simulink library "IP_MASTER_backup20190216"  (Simulink 8.6)
settings: Solver=ode45  StartTime=0.0  StopTime=10.0  RelTol=1e-3
libraries: cdsFilt x19, cdsEpicsOut x14, cdsFiltCtrl x12, cdsTP x6, cdsMuxMatrix x3, cdsEpicsIn x3, cdsFunctionCall x1, SIXOSEM_F_WD_AC_MASTER x1, SIXOSEM_F_STAGE_MASTER x1
(part 1 of 4)
settings Model: Creator=controls  LastModifiedBy=controls

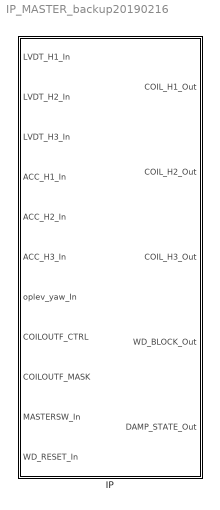
== system IP_MASTER_backup20190216 ==
  IP : Subsystem

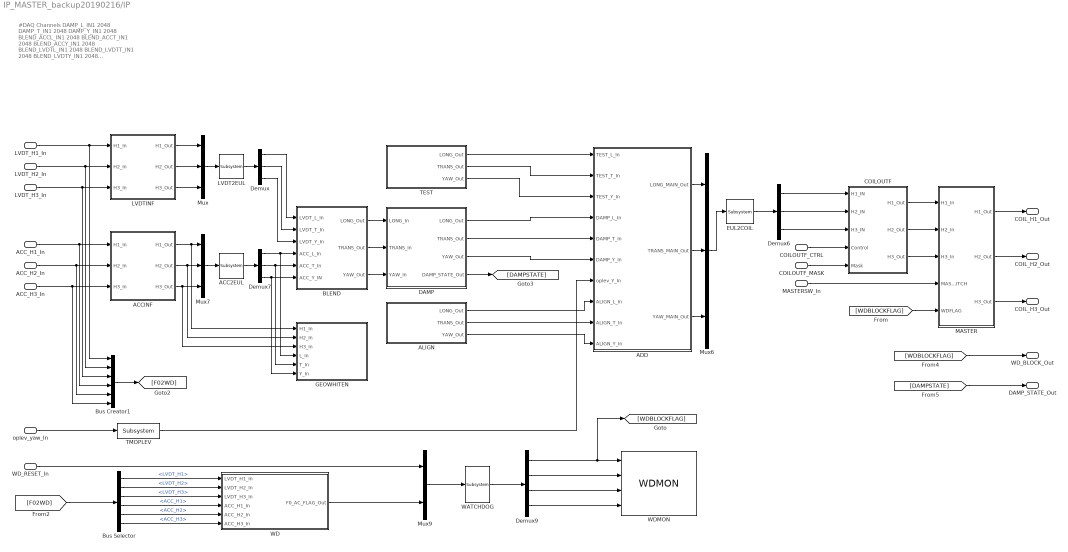
== system IP_MASTER_backup20190216/IP ==
  note: #DAQ Channels
      | DAMP_L_IN1 2048
      | DAMP_T_IN1 2048
      | DAMP_Y_IN1 2048
      | BLEND_ACCL_IN1 2048
      | BLEND_ACCT_IN1 2048
      | BLEND_ACCY_IN1 2048
      | BLEND_LVDTL_IN1 2048
      | BLEND_LVDTT_IN1 2048
      | BLEND_LVDTY_IN1 2048
      | GEOWHITEN_L_OUT 2048
      | GEOWHITEN_T_OUT 2048
      | GEOWHITEN_Y_OUT 2048
  LVDT_H1_In : Inport
  LVDT_H2_In : Inport  Port=2
  LVDT_H3_In : Inport  Port=3
  ACC_H1_In : Inport  Port=4
  ACC_H2_In : Inport  Port=5
  ACC_H3_In : Inport  Port=6
  oplev_yaw_In : Inport  Port=7
  COILOUTF_CTRL : Inport  Port=8
  COILOUTF_MASK : Inport  Port=9
  MASTERSW_In : Inport  Port=10
  WD_RESET_In : Inport  Port=11
  ACC2EUL : cdsMuxMatrix/Subsystem  Tag=cdsMuxMatrix  Description=|
      | ADL=SUS_INMATRIX.adl
      | SCRIPT=generate_KisselButton.py 4 5 #CHANNEL# > #TARGET_DIR#/#FULL_PART_NAME#_KB.adl
      settings: AttributesFormatString=%<Tag>
  ACCINF : Subsystem
  ADD : Subsystem
  ALIGN : Subsystem
  BLEND : Subsystem
  Bus Creator1 : BusCreator  Inputs='LVDT_H1','LVDT_H2','LVDT_H3','ACC_H1','ACC_H2','ACC_H3'
  Bus Selector : BusSelector  OutputSignals=LVDT_H1,LVDT_H2,LVDT_H3,ACC_H1,ACC_H2,ACC_H3
  COILOUTF : Subsystem
  DAMP : Subsystem
  Demux : Demux  Outputs=3
  Demux6 : Demux  Outputs=3
  Demux7 : Demux  Outputs=3
  Demux9 : Demux
  EUL2COIL : cdsMuxMatrix/Subsystem  Tag=cdsMuxMatrix  Description=|
      | ADL=SUS_INMATRIX.adl
      | SCRIPT=generate_KisselButton.py 4 5 #CHANNEL# > #TARGET_DIR#/#FULL_PART_NAME#_KB.adl
      settings: AttributesFormatString=%<Tag>
  GEOWHITEN : Subsystem
  LVDT2EUL : cdsMuxMatrix/Subsystem  Tag=cdsMuxMatrix  Description=|
      | ADL=SUS_INMATRIX.adl
      | SCRIPT=generate_KisselButton.py 4 5 #CHANNEL# > #TARGET_DIR#/#FULL_PART_NAME#_KB.adl
      settings: AttributesFormatString=%<Tag>
  LVDTINF : Subsystem
  MASTER : Subsystem
  Mux : Mux  Inputs=3
  Mux6 : Mux  Inputs=3
  Mux7 : Mux  Inputs=3
  Mux9 : Mux  Inputs=2
  TEST : Subsystem
  TMOPLEV : cdsFilt/Subsystem  Tag=cdsFilt  Description=|
      | Purpose:                                                                                                                                                                                                                                  
      | Standard CDS IIR filter module.                                                                                                                                                                                                           
      |                                                                                                                                                                                                                                           
      | Operation:                                                                                                                                                                                                                                
      | Consists of 10 second order section IIR filters, plus a ramped gain stage. In FE code, also provides pre-defined test points and excitation channel inputs. The filter coefficients are defined in the LIGO system using the 'foton' tool.
      |                                                                                                                                                                                                                                           
      | Usage:                                                                                                                                                                                                                                    
      | Name the part with the desired filter module name.
      settings: AttributesFormatString=%<Tag>
  WATCHDOG : cdsFunctionCall/Subsystem  Tag=cdsFunctionCall  Description=inline OSEMWATCHDOG /opt/rtcds/userapps/release/vis/common/src/WATCHDOG.c
      settings: AttributesFormatString=%<Tag>\n%<Description>
  WD : Subsystem
  WDMON : SIXOSEM_F_STAGE_MASTER/SIXOSEM_F_STAGE_MASTER/WDMON
  COIL_H1_Out : Outport
  COIL_H2_Out : Outport  Port=2
  COIL_H3_Out : Outport  Port=3
  WD_BLOCK_Out : Outport  Port=4
  DAMP_STATE_Out : Outport  Port=5
  wires:
  LVDTINF/1(H1_Out) -> Mux/1
  LVDTINF/2(H2_Out) -> Mux/2
  LVDTINF/3(H3_Out) -> Mux/3
  Mux/1 -> LVDT2EUL/1
  LVDT2EUL/1 -> Demux/1
  Mux7/1 -> ACC2EUL/1
  ACCINF/1(H1_Out) -> GEOWHITEN/1(H1_In), Mux7/1
  ACCINF/3(H3_Out) -> GEOWHITEN/3(H3_In), Mux7/3
  ACCINF/2(H2_Out) -> GEOWHITEN/2(H2_In), Mux7/2
  ACC2EUL/1 -> Demux7/1
  Demux/1 -> BLEND/1(LVDT_L_In)
  Demux/2 -> BLEND/2(LVDT_T_In)
  Demux/3 -> BLEND/3(LVDT_Y_In)
  Demux7/1 -> GEOWHITEN/4(L_In), BLEND/4(ACC_L_In)
  Demux7/2 -> GEOWHITEN/5(T_In), BLEND/5(ACC_T_In)
  Demux7/3 -> GEOWHITEN/6(Y_In), BLEND/6(ACC_Y_IN)
  ADD/1(LONG_MAIN_Out) -> Mux6/1
  ADD/2(TRANS_MAIN_Out) -> Mux6/2
  ADD/3(YAW_MAIN_Out) -> Mux6/3
  Mux6/1 -> EUL2COIL/1
  EUL2COIL/1 -> Demux6/1
  Demux6/1 -> COILOUTF/1(H1_IN)
  Demux6/2 -> COILOUTF/2(H2_IN)
  Demux6/3 -> COILOUTF/3(H3_IN)
  MASTER/1(H1_Out) -> COIL_H1_Out/1
  MASTER/2(H2_Out) -> COIL_H2_Out/1
  MASTER/3(H3_Out) -> COIL_H3_Out/1
  COILOUTF/1(H1_Out) -> MASTER/1(H1_In)
  COILOUTF/2(H2_Out) -> MASTER/2(H2_In)
  COILOUTF/3(H3_Out) -> MASTER/3(H3_In)
  MASTERSW_In/1 -> MASTER/4(MASTERSWITCH)
  WD_RESET_In/1 -> Mux9/1
  WD/1(F0_AC_FLAG_Out) -> Mux9/2
  [F02WD] -> Bus Selector/1
  Bus Selector/1 -> WD/1(LVDT_H1_In)  "<LVDT_H1>"
  Bus Selector/2 -> WD/2(LVDT_H2_In)  "<LVDT_H2>"
  Bus Selector/3 -> WD/3(LVDT_H3_In)  "<LVDT_H3>"
  Bus Selector/4 -> WD/4(ACC_H1_In)  "<ACC_H1>"
  Bus Selector/6 -> WD/6(ACC_H3_In)  "<ACC_H3>"
  Bus Selector/5 -> WD/5(ACC_H2_In)  "<ACC_H2>"
  Demux9/1 -> [WDBLOCKFLAG], WDMON/1
  Demux9/2 -> WDMON/2
  Demux9/3 -> WDMON/3
  Demux9/4 -> WDMON/4
  Mux9/1 -> WATCHDOG/1
  WATCHDOG/1 -> Demux9/1
  LVDT_H1_In/1 -> Bus Creator1/1, LVDTINF/1(H1_In)
  LVDT_H2_In/1 -> Bus Creator1/2, LVDTINF/2(H2_In)
  LVDT_H3_In/1 -> Bus Creator1/3, LVDTINF/3(H3_In)
  ACC_H1_In/1 -> Bus Creator1/4, ACCINF/1(H1_In)
  ACC_H2_In/1 -> Bus Creator1/5, ACCINF/2(H2_In)
  ACC_H3_In/1 -> Bus Creator1/6, ACCINF/3(H3_In)
  Bus Creator1/1 -> [F02WD]
  [WDBLOCKFLAG] -> MASTER/5(WDFLAG)
  BLEND/1(LONG_Out) -> DAMP/1(LONG_In)
  BLEND/2(TRANS_Out) -> DAMP/2(TRANS_In)
  BLEND/3(YAW_Out) -> DAMP/3(YAW_In)
  DAMP/4(DAMP_STATE_Out) -> [DAMPSTATE]
  TEST/1(LONG_Out) -> ADD/1(TEST_L_In)
  TEST/2(TRANS_Out) -> ADD/2(TEST_T_In)
  TEST/3(YAW_Out) -> ADD/3(TEST_Y_In)
  DAMP/1(LONG_Out) -> ADD/4(DAMP_L_In)
  DAMP/2(TRANS_Out) -> ADD/5(DAMP_T_In)
  DAMP/3(YAW_Out) -> ADD/6(DAMP_Y_In)
  COILOUTF_CTRL/1 -> COILOUTF/4(Control)
  COILOUTF_MASK/1 -> COILOUTF/5(Mask)
  [WDBLOCKFLAG] -> WD_BLOCK_Out/1
  [DAMPSTATE] -> DAMP_STATE_Out/1
  oplev_yaw_In/1 -> TMOPLEV/1
  TMOPLEV/1 -> ADD/7(oplev_Y_In)
  ALIGN/1(LONG_Out) -> ADD/8(ALIGN_L_In)
  ALIGN/2(TRANS_Out) -> ADD/9("ALIGN_T_In ")
  ALIGN/3(YAW_Out) -> ADD/10(ALIGN_Y_In)

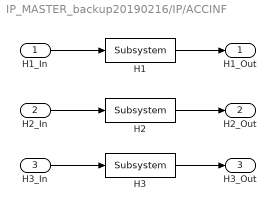
== system IP_MASTER_backup20190216/IP/ACCINF ==
  H1_In : Inport
  H2_In : Inport  Port=2
  H3_In : Inport  Port=3
  H1 : cdsFilt/Subsystem  Tag=cdsFilt  Description=|
      | Purpose:                                                                                                                                                                                                                                  
      | Standard CDS IIR filter module.                                                                                                                                                                                                           
      |                                                                                                                                                                                                                                           
      | Operation:                                                                                                                                                                                                                                
      | Consists of 10 second order section IIR filters, plus a ramped gain stage. In FE code, also provides pre-defined test points and excitation channel inputs. The filter coefficients are defined in the LIGO system using the 'foton' tool.
      |                                                                                                                                                                                                                                           
      | Usage:                                                                                                                                                                                                                                    
      | Name the part with the desired filter module name.
      settings: AttributesFormatString=%<Tag>
  H2 : cdsFilt/Subsystem  Tag=cdsFilt  Description=|
      | Purpose:                                                                                                                                                                                                                                  
      | Standard CDS IIR filter module.                                                                                                                                                                                                           
      |                                                                                                                                                                                                                                           
      | Operation:                                                                                                                                                                                                                                
      | Consists of 10 second order section IIR filters, plus a ramped gain stage. In FE code, also provides pre-defined test points and excitation channel inputs. The filter coefficients are defined in the LIGO system using the 'foton' tool.
      |                                                                                                                                                                                                                                           
      | Usage:                                                                                                                                                                                                                                    
      | Name the part with the desired filter module name.
      settings: AttributesFormatString=%<Tag>
  H3 : cdsFilt/Subsystem  Tag=cdsFilt  Description=|
      | Purpose:                                                                                                                                                                                                                                  
      | Standard CDS IIR filter module.                                                                                                                                                                                                           
      |                                                                                                                                                                                                                                           
      | Operation:                                                                                                                                                                                                                                
      | Consists of 10 second order section IIR filters, plus a ramped gain stage. In FE code, also provides pre-defined test points and excitation channel inputs. The filter coefficients are defined in the LIGO system using the 'foton' tool.
      |                                                                                                                                                                                                                                           
      | Usage:                                                                                                                                                                                                                                    
      | Name the part with the desired filter module name.
      settings: AttributesFormatString=%<Tag>
  H1_Out : Outport
  H2_Out : Outport  Port=2
  H3_Out : Outport  Port=3
  wires:
  H1_In/1 -> H1/1
  H1/1 -> H1_Out/1
  H2_In/1 -> H2/1
  H2/1 -> H2_Out/1
  H3_In/1 -> H3/1
  H3/1 -> H3_Out/1

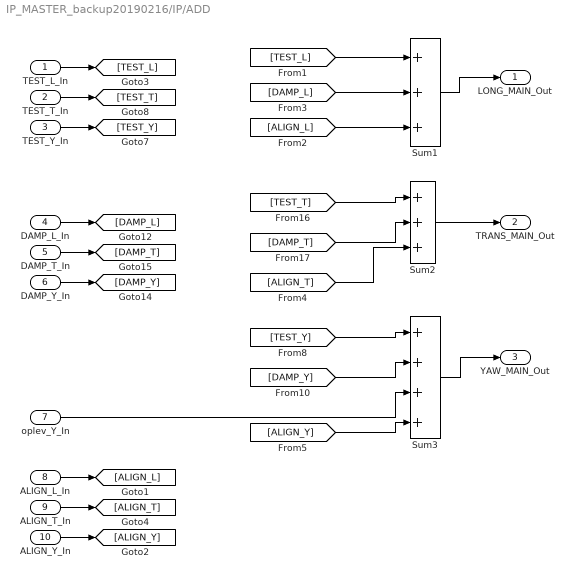
== system IP_MASTER_backup20190216/IP/ADD ==
  TEST_L_In : Inport
  TEST_T_In : Inport  Port=2
  TEST_Y_In : Inport  Port=3
  DAMP_L_In : Inport  Port=4
  DAMP_T_In : Inport  Port=5
  DAMP_Y_In : Inport  Port=6
  oplev_Y_In : Inport  Port=7
  ALIGN_L_In : Inport  Port=8
  "ALIGN_T_In " : Inport  Port=9
  ALIGN_Y_In : Inport  Port=10
  Sum1 : Sum  Inputs=+++
  Sum2 : Sum  Inputs=+++
  Sum3 : Sum  Inputs=++++
  LONG_MAIN_Out : Outport
  TRANS_MAIN_Out : Outport  Port=2
  YAW_MAIN_Out : Outport  Port=3
  wires:
  Sum1/1 -> LONG_MAIN_Out/1
  TEST_L_In/1 -> [TEST_L]
  TEST_T_In/1 -> [TEST_T]
  TEST_Y_In/1 -> [TEST_Y]
  DAMP_L_In/1 -> [DAMP_L]
  DAMP_T_In/1 -> [DAMP_T]
  DAMP_Y_In/1 -> [DAMP_Y]
  Sum2/1 -> TRANS_MAIN_Out/1
  Sum3/1 -> YAW_MAIN_Out/1
  [DAMP_L] -> Sum1/2
  [TEST_L] -> Sum1/1
  [TEST_T] -> Sum2/1
  [DAMP_T] -> Sum2/2
  [TEST_Y] -> Sum3/1
  [DAMP_Y] -> Sum3/2
  oplev_Y_In/1 -> Sum3/3
  ALIGN_L_In/1 -> [ALIGN_L]
  "ALIGN_T_In "/1 -> [ALIGN_T]
  ALIGN_Y_In/1 -> [ALIGN_Y]
  [ALIGN_L] -> Sum1/3
  [ALIGN_T] -> Sum2/3
  [ALIGN_Y] -> Sum3/4

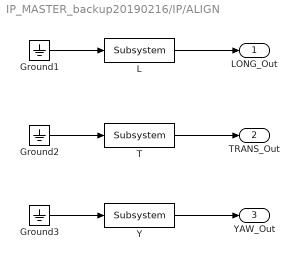
== system IP_MASTER_backup20190216/IP/ALIGN ==
  Ground1 : Ground
  Ground2 : Ground
  Ground3 : Ground
  L : cdsFilt/Subsystem  Tag=cdsFilt  Description=|
      | Purpose:                                                                                                                                                                                                                                  
      | Standard CDS IIR filter module.                                                                                                                                                                                                           
      |                                                                                                                                                                                                                                           
      | Operation:                                                                                                                                                                                                                                
      | Consists of 10 second order section IIR filters, plus a ramped gain stage. In FE code, also provides pre-defined test points and excitation channel inputs. The filter coefficients are defined in the LIGO system using the 'foton' tool.
      |                                                                                                                                                                                                                                           
      | Usage:                                                                                                                                                                                                                                    
      | Name the part with the desired filter module name.
      settings: AttributesFormatString=%<Tag>
  T : cdsFilt/Subsystem  Tag=cdsFilt  Description=|
      | Purpose:                                                                                                                                                                                                                                  
      | Standard CDS IIR filter module.                                                                                                                                                                                                           
      |                                                                                                                                                                                                                                           
      | Operation:                                                                                                                                                                                                                                
      | Consists of 10 second order section IIR filters, plus a ramped gain stage. In FE code, also provides pre-defined test points and excitation channel inputs. The filter coefficients are defined in the LIGO system using the 'foton' tool.
      |                                                                                                                                                                                                                                           
      | Usage:                                                                                                                                                                                                                                    
      | Name the part with the desired filter module name.
      settings: AttributesFormatString=%<Tag>
  Y : cdsFilt/Subsystem  Tag=cdsFilt  Description=|
      | Purpose:                                                                                                                                                                                                                                  
      | Standard CDS IIR filter module.                                                                                                                                                                                                           
      |                                                                                                                                                                                                                                           
      | Operation:                                                                                                                                                                                                                                
      | Consists of 10 second order section IIR filters, plus a ramped gain stage. In FE code, also provides pre-defined test points and excitation channel inputs. The filter coefficients are defined in the LIGO system using the 'foton' tool.
      |                                                                                                                                                                                                                                           
      | Usage:                                                                                                                                                                                                                                    
      | Name the part with the desired filter module name.
      settings: AttributesFormatString=%<Tag>
  LONG_Out : Outport
  TRANS_Out : Outport  Port=2
  YAW_Out : Outport  Port=3
  wires:
  T/1 -> TRANS_Out/1
  L/1 -> LONG_Out/1
  Ground1/1 -> L/1
  Ground2/1 -> T/1
  Y/1 -> YAW_Out/1
  Ground3/1 -> Y/1
